simulink model "AutonomosBike_fuzzy (2)"  (R2019a)
settings: Solver=VariableStepAuto  StartTime=0.0  StopTime=1000  RelTol=1e-3
libraries: fuzblock x1
settings Model: Creator=Nidia R  LastModifiedBy=Nidia R

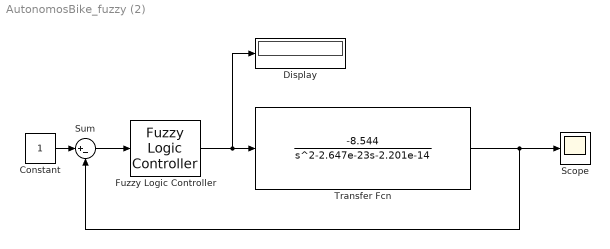
== system AutonomosBike_fuzzy (2) ==
  Constant : Constant
  Display : Display
  Fuzzy Logic Controller : fuzblock/Fuzzy Logic  Controller  FIS='FussyBikeA.fis'  OutputSampleNumber=101  DataType=double  FuzzifiedInputs=off  RuleFiringStrengths=off  RuleOutputs=off  AggregatedOutputs=off  SimulateUsing=Interpreted execution  OutOfRangeInputValueMessage=warning  NoRuleFiredMessage=warning  EmptyOutputFuzzySetMessage=warning
  Scope : Scope
  Sum : Sum  Inputs=|+-
  Transfer Fcn : TransferFcn  Numerator=[-8.544]  Denominator=[1 -2.647e-23 -2.201e-14]
  wires:
  Fuzzy Logic Controller/1 -> Display/1, Transfer Fcn/1
  Transfer Fcn/1 -> Sum/2, Scope/1
  Constant/1 -> Sum/1
  Sum/1 -> Fuzzy Logic Controller/1
